simulink model "sf_demo"  (Simulink 6.4)
settings: Solver=FixedStepDiscrete  StartTime=0.0  StopTime=20  FixedStep=0.5  RelTol=1e-3
PreLoadFcn:
  | if exist('tl_preloadfcn','file'), tl_preloadfcn(gcs,95); end
PostLoadFcn:
  | if exist('tl_postloadfcn','file'), tl_postloadfcn(gcs,95); end
InitFcn:
  | if exist('tlds_start','file'), tlds_start(gcs); end
undefined symbols (not defined in the file or in its folder): built, Gain, in, Sum
libraries: tllib x18, simulink x1
PreSaveFcn:
  | if exist('tl_presavefcn','file'), tl_presavefcn(gcs); end
settings Model: LastModifiedBy=hilgers  ExtModeTrigMode=oneshot  ExtModeArmWhenConnect=off  BufferReuse=off  DS_PROJECTFILE=sf_demo.dd  TL_MAIN_DATA=struct('codeopt',struct('target',['Generic ANSI-C'],'optlevel',0,'sfbitfields',1,'limidentlength',1,'decimals',0,'assembler',1,'sections',1,'separatesearch',0,'cleancode',0,'optimizedbooltype',1,'inliningthreshold',5,'linebreaklimit',100,'stateactcodinglimit',5,'functionsfor64bitops',1,'globalbitfields',0,'sharefunctions',0,'noinitstozero',0,'keepsaturation',0,'extvarsharing',0,'outputstylefile','cconfig.xml','rootstylesheet','TL_CSourceCodeSS.xsl'),'frameopt',struct('exectime',1,'stacksize',1,'mexargs','','simconfig',['default EVM'],'targettimeout',1,'tcargs',''),'logopt',struct('plotinterval',0.1,'globalloggingmode',1),'date',732484.795619213,'asapscript','asap2_all_in_one','docscript','tldoc_default','maxnumsimulations',10,'export',struct('directory','.\export','sysfiles',1,'docfiles',0,'tools',0),'codecoveragelevel',0,'rtos',struct('enablemultirate',0,'currentrtos',['generic RTOS'],'autopriority',0,'autoinitalarm',1,'alarminitwithrestart',1,'alarmactivationkind',1,'alarmstartoffset',0))  TL_MODEL_COMMENT=This model implements a simple state machine.
settings DataIOCC: LimitDataPoints=off
settings OptimizationCC: BlockReduction=off  BooleanDataType=off  OptimizeBlockIOStorage=off  BufferReuse=off  ExpressionFolding=off  LocalBlockOutputs=off
settings DebuggingCC: SolverPrmCheckMsg=none  StrictBusMsg=None
settings HardwareCC: TargetEndianess=LittleEndian  TargetHWDeviceType=MATLAB Host  ProdEqTarget=off

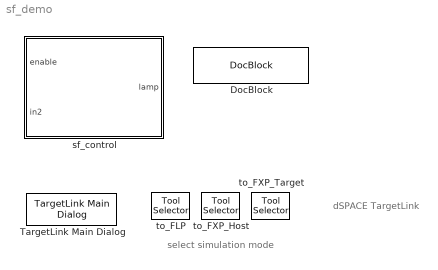
== system sf_demo ==
  note: select simulation mode
  note: dSPACE TargetLink
  DocBlock : simulink/Model-Wide Utilities/DocBlock  SystemSampleTime=-1  DocumentType=Text
  TargetLink Main Dialog : tllib/TargetLink Main Dialog  SystemSampleTime=-1  flp_block=none
  sf_control : Subsystem  Tag=TargetLink Simulation Frame
      settings: CopyFcn=if exist('tl_copyfcn','file'), tl_copyfcn(gcbh); end  NameChangeFcn=if exist('tl_framenamechangefcn','file'), tl_framenamechangefcn(gcbh); end  OpenFcn=if exist('open_tlsubsystem','file'), open_tlsubsystem(gcbh); end
      mask Type: TL_SimFrame
      mask Display: disp('TargetLink\nModel-\nin-the-loop\nmode')
  to_FLP : tllib/Tool Selector  Description=MIL\nmode  SystemSampleTime=-1  data=struct('date',732004.630535799)  flp_block=none
  to_FXP_Host : tllib/Tool Selector  Description=SIL\nmode  SystemSampleTime=-1  data=struct('date',732004.630535914)  flp_block=none
  to_FXP_Target : tllib/Tool Selector  Description=PIL\nmode  SystemSampleTime=-1  data=struct('date',732004.63053603)  flp_block=none

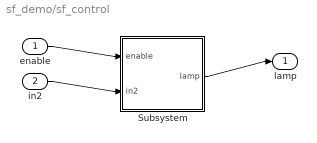
== system sf_demo/sf_control ==
  enable : Inport  PortDimensions=1  SampleTime=0.5  DataType=Specify via dialog  OutDataType=osc_int16
  in2 : Inport  Port=2  PortDimensions=1  SampleTime=0.5  DataType=Specify via dialog  OutDataType=osc_uint32
  Subsystem : Subsystem
      settings: OpenFcn=warndlg(get_param(gcb,'MaskHelp'),'Serious Warning');
      mask Type: TL_Enable
      mask Help: This subsystem keeps the TargetLink subsystem (subsystem with TargetLink blocks for production code generation), and is needed for the TargetLink simulation frame to work properly. DO NOT DELETE OR MODIFY IT!
  lamp : Outport
  wires:
  enable/1 -> Subsystem/1(enable)
  in2/1 -> Subsystem/2(in2)
  Subsystem/1(lamp) -> lamp/1

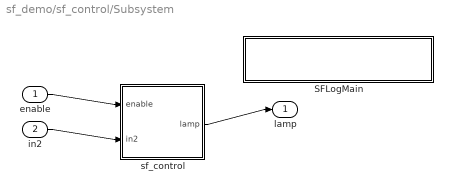
== system sf_demo/sf_control/Subsystem ==
  enable : Inport  PortDimensions=1  SampleTime=0.5  DataType=Specify via dialog  OutDataType=osc_int16
  in2 : Inport  Port=2  PortDimensions=1  SampleTime=0.5  DataType=Specify via dialog  OutDataType=osc_uint32
  SFLogMain : Subsystem
      mask Type: TL_StateflowLoggingMain
      mask Display:
      | plot([0 0 1 1 0 0 1 1 0],[0 1 1 0 0 0.05 0.05 0.95 0.95]);
      | disp('Stateflow Logging Main\nDO NOT DELETE')
  sf_control : Subsystem  Tag=MIL Subsystem  Description=a
      settings: CopyFcn=if exist('tl_copyfcn','file'), tl_copyfcn(gcbh); end  NameChangeFcn=if exist('tl_namechangefcn','file'), tl_namechangefcn(gcbh); end  DestroyFcn=if exist('update_tl_main_dlg','file'), update_tl_main_dlg('TL_subs_display'); end
  lamp : Outport
  wires:
  enable/1 -> sf_control/1(enable)
  in2/1 -> sf_control/2(in2)
  sf_control/1(lamp) -> lamp/1

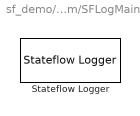
== system sf_demo/sf_control/Subsystem/SFLogMain ==
  Stateflow Logger : tllib/Extras/Stateflow Logger  data=struct('date',732004.630533947)  sflogparam=struct('charts',163,'sfblocks',{{'sf_demo/sf_control/Subsystem/sf_control/SF_TEST_B'}},'machines',162,'globallogopt',1,'modelname','sf_demo','debugmodeactive',1)  flp_block=tldummylib/Stateflow Logger

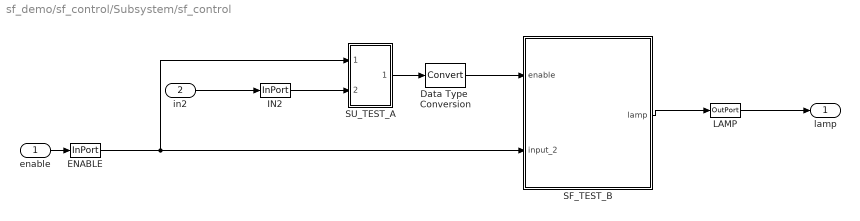
== system sf_demo/sf_control/Subsystem/sf_control ==
  enable : Inport  PortDimensions=1  SampleTime=0.5  DataType=Specify via dialog  OutDataType=osc_int16
      settings: CopyFcn=if exist('tl_check_ports','file'), tl_check_ports(gcbh); end  NameChangeFcn=if exist('tl_check_ports','file'), tl_check_ports(gcbh); end
  in2 : Inport  Port=2  PortDimensions=1  SampleTime=0.5  DataType=Specify via dialog  OutDataType=osc_uint32
      settings: CopyFcn=if exist('tl_check_ports','file'), tl_check_ports(gcbh); end  NameChangeFcn=if exist('tl_check_ports','file'), tl_check_ports(gcbh); end
  Data Type  Conversion : DataTypeConversion  OutDataTypeMode=Specify via dialog  OutDataType=osc_boolean  SaturateOnIntegerOverflow=on  RndMeth=Zero
  ENABLE : tllib/InPort  SystemSampleTime=-1  data=struct('logdata',struct('maxnumvals',4096,'plotchannels',1,'channels',1,'loggingmode',1),'output',struct('width',1,'name','$S_$B','unit','','type','Int8','offset',0,'max',1,'min',0,'freeze',1,'lsb',1,'arb',0,'class','FCN_ARG','address','','show',0,'description','','autoscalingmode',1,'lowerheadroom',1,'upperheadroom',1,'headroomunit','bit','variable','','scaling','','keepdatatype',1,'castoutput',0),'date',732458.608520498,'virtual',1,'message',struct('name','','component','','accessor',''),'scalingvalid',0)  flp_block=none
  IN2 : tllib/InPort  SystemSampleTime=-1  data=struct('logdata',struct('maxnumvals',4096,'plotchannels',1,'channels',1,'loggingmode',1),'output',struct('width',1,'name','$S_$B','unit','','type','Int8','offset',0,'max',1,'min',0,'freeze',1,'lsb',1,'arb',0,'class','FCN_ARG','address','','show',0,'description','','autoscalingmode',1,'lowerheadroom',1,'upperheadroom',1,'headroomunit','bit','variable','','scaling','','keepdatatype',1,'castoutput',0),'date',732463.617900926,'virtual',1,'message',struct('name','','component','','accessor',''),'scalingvalid',0)  flp_block=none
  LAMP : tllib/OutPort  SystemSampleTime=-1  data=struct('comment',struct('text','','placement',1),'logdata',struct('maxnumvals',inf,'plotchannels',1,'channels',1,'loggingmode',1),'output',struct('width',1,'name','$S_$B','unit','','type','Int8','offset',0,'max',1,'min',0,'freeze',1,'lsb',1,'arb',0,'class','FCN_RETURN','address','','checkmin',0,'checkmax',0,'show',0,'description','','autoscalingmode',1,'lowerheadroom',1,'upperheadroom',1,'headroomunit','bit','variable','','scaling','','keepdatatype',1,'castoutput',0),'date',732463.632425845,'virtual',1,'message',struct('name','','component',''),'scalingvalid',0)  flp_block=none
  SF_TEST_B : Stateflow chart
  SU_TEST_A : Subsystem  TreatAsAtomicUnit=on
  lamp : Outport
      settings: CopyFcn=if exist('tl_check_ports','file'), tl_check_ports(gcbh); end  NameChangeFcn=if exist('tl_check_ports','file'), tl_check_ports(gcbh); end
  wires:
  SF_TEST_B/1(lamp) -> LAMP/1
  LAMP/1 -> lamp/1
  enable/1 -> ENABLE/1
  in2/1 -> IN2/1
  ENABLE/1 -> SU_TEST_A/1(In1), SF_TEST_B/2(input_2)
  IN2/1 -> SU_TEST_A/2(In2)
  SU_TEST_A/1(Out1) -> Data Type  Conversion/1
  Data Type  Conversion/1 -> SF_TEST_B/1(enable)

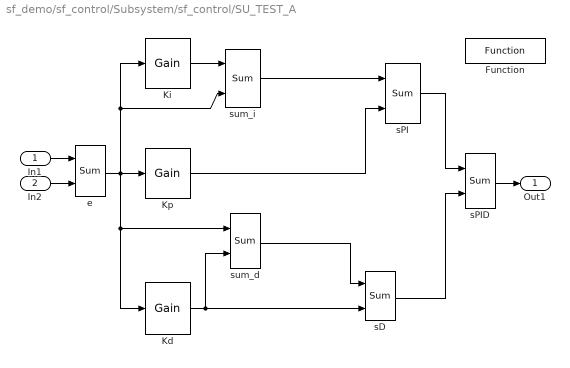
== system sf_demo/sf_control/Subsystem/sf_control/SU_TEST_A ==
  In1 : Inport  DataType=Specify via dialog  OutDataType=osc_int16
  In2 : Inport  Port=2  DataType=Specify via dialog  OutDataType=osc_uint32
  Function : tllib/Function  SystemSampleTime=-1  data=struct('revisionNumber',9,'description','','stepfunctionname','$S_$B','stepfunctionclass','default','forcerestartfunction',0,'restartfunctionname','RESTART_$S_$B','restartfunctionclass','default','forceinitfunction',0,'initfunctionname','INIT_$S_$B','initfunctionclass','default','forcetermfunction',0,'termfunctionname','TERM_$S_$B','termfunctionclass','default','subsystemid','default','forcereuse',0,'linkfile',0,'functionarglist',{{}},'unscaledarguments',0,'scalingpropagation',{{}},'incrcodegen',0,'ownedmodules',{{}},'destination','','addtestframe',0,'simmode',1,'codecomment','','codefile','','codecoveragelevel',0)  flp_block=tldummylib/Function
  Kd : tllib/Gain  Tag="Gain block of the dSPACE Fixed Point Code Generation Environment.      \\n                                                                       \\n signal is equal to the product of the input signal and the gain value:\\n\t\ty = G u"  SystemSampleTime=-1  data=struct('gain',struct('value','4','type','UInt8','lsb',2^-5,'offset',0,'min',NaN,'max',NaN,'arb',0,'freeze',1,'width',1,'scalar',0,'name','P_$D','class','CAL','address','','unit','','description','','tolerance',1,'variable','','scaling','','keepdatatype',1),'logdata',struct('maxnumvals',inf,'plotchannels',1,'channels',1,'loggingmode',3),'output',struct('type','Int16','lsb',2^-15,'offset',0,'max',NaN,'min',NaN,'checkmin',0,'checkmax',0,'arb',0,'freeze',1,'width',1,'name','$S_$B','show',0,'class','default','address','','unit','','description','','autoscalingmode',1,'lowerheadroom',1,'upperheadroom',1,'headroomunit','bit','variable','','scaling','','keepdatatype',1,'castoutput',0),'comment',struct('text','','placement',1),'date',732457.587188403,'scalingvalid',0)  gain=4  flp_block=built-in/Gain  help=Gain block of dSPACE TargetLink.\n\nOutput signal is equal to the product of the input signal and the gain value:\n\t\ty = G u
  Ki : tllib/Gain  SystemSampleTime=-1  data=struct('gain',struct('value','0.2','type','UInt8','lsb',2^-10,'offset',0,'min',NaN,'max',NaN,'arb',0,'freeze',1,'width',1,'scalar',0,'name','P_$D','class','CAL','address','','unit','','description','','tolerance',1,'variable','','scaling','','keepdatatype',1),'logdata',struct('maxnumvals',inf,'plotchannels',[],'channels',1,'loggingmode',3),'output',struct('type','Int16','lsb',2^-20,'offset',0,'max',NaN,'min',NaN,'checkmin',0,'checkmax',0,'arb',0,'freeze',1,'width',1,'name','$S_$B','show',0,'class','default','address','','unit','','description','','autoscalingmode',1,'lowerheadroom',1,'upperheadroom',1,'headroomunit','bit','variable','','scaling','','keepdatatype',1,'castoutput',0),'comment',struct('text','','placement',1),'date',732457.586778785,'scalingvalid',0)  gain=0.2  flp_block=built-in/Gain  help=Gain block of dSPACE TargetLink.\n\nOutput signal is equal to the product of the input signal and the gain value:\n\t\ty = G u
  Kp : tllib/Gain  Tag="Gain block of the dSPACE Fixed Point Code Generation Environment.      \\n                                                                       \\n signal is equal to the product of the input signal and the gain value:\\n\t\ty = G u"  SystemSampleTime=-1  data=struct('gain',struct('value','1.2','type','UInt8','lsb',2^-7,'offset',0,'min',NaN,'max',NaN,'arb',0,'freeze',1,'width',1,'scalar',0,'name','P_$D','class','CAL','address','','unit','','description','','tolerance',1,'variable','','scaling','','keepdatatype',1),'logdata',struct('maxnumvals',inf,'plotchannels',[],'channels',1,'loggingmode',3),'output',struct('type','Int16','lsb',2^-17,'offset',0,'max',NaN,'min',NaN,'checkmin',0,'checkmax',0,'arb',0,'freeze',1,'width',1,'name','$S_$B','show',0,'class','default','address','','unit','','description','','autoscalingmode',1,'lowerheadroom',1,'upperheadroom',1,'headroomunit','bit','variable','','scaling','','keepdatatype',1,'castoutput',0),'comment',struct('text','','placement',1),'date',732457.587011169,'scalingvalid',0)  gain=1.2  flp_block=built-in/Gain  help=Gain block of dSPACE TargetLink.\n\nOutput signal is equal to the product of the input signal and the gain value:\n\t\ty = G u
  e : tllib/Sum  data=struct('logdata',struct('maxnumvals',inf,'plotchannels',1,'channels',1,'loggingmode',1),'output',struct('type','Int16','lsb',2^-18,'offset',0,'max',NaN,'min',NaN,'checkmin',1,'checkmax',1,'arb',0,'freeze',1,'width',1,'name','$S_$B','show',0,'class','default','address','','unit','','description','','autoscalingmode',1,'lowerheadroom',1,'upperheadroom',1,'headroomunit','bit','variable','','scaling','','keepdatatype',1,'castoutput',0),'inputs','+-','comment',struct('text','','placement',1),'date',732457.596463576,'scalingvalid',0)  flp_block=built-in/Sum  help=Sum block of dSPACE TargetLink.\n\nOutput signal is equal to the sum of the input signals.\nThe list of signs is specified according to conventions for Simulink Sum blocks.
  sD : tllib/Sum  Tag="Sum block of the dSPACE Fixed Point Code Generation Environment.\\n                                                                \\nOutput signal is equal to the sum of the two input signals:     \\n                                                                \\n\t\ty = u1 - u2"  data=struct('logdata',struct('maxnumvals',inf,'plotchannels',1,'channels',1,'loggingmode',3),'output',struct('type','Int16','lsb',2^-15,'offset',0,'max',NaN,'min',NaN,'checkmin',0,'checkmax',0,'arb',0,'freeze',1,'width',1,'name','$S_$B','show',0,'class','default','address','','unit','','description','','autoscalingmode',1,'lowerheadroom',1,'upperheadroom',1,'headroomunit','bit','variable','','scaling','','keepdatatype',1,'castoutput',0),'inputs','++','comment',struct('text','','placement',1),'date',732004.633502326,'scalingvalid',0)  flp_block=built-in/Sum  help=Sum block of dSPACE TargetLink.\n\nOutput signal is equal to the sum of the input signals.\nThe list of signs is specified according to conventions for Simulink Sum blocks.
  sPI : tllib/Sum  Tag="Sum block of the dSPACE Fixed Point Code Generation Environment.\\n                                                                \\nOutput signal is equal to the sum of the two input signals:     \\n                                                                \\n\t\ty = u1 - u2"  data=struct('logdata',struct('maxnumvals',inf,'plotchannels',[],'channels',1,'loggingmode',3),'output',struct('type','Int16','lsb',2^-17,'offset',0,'max',NaN,'min',NaN,'checkmin',0,'checkmax',0,'arb',0,'freeze',1,'width',1,'name','$S_$B','show',0,'class','default','address','','unit','','description','','autoscalingmode',1,'lowerheadroom',1,'upperheadroom',1,'headroomunit','bit','variable','','scaling','','keepdatatype',1,'castoutput',0),'inputs','++','comment',struct('text','','placement',1),'date',732004.633503032,'scalingvalid',0)  flp_block=built-in/Sum  help=Sum block of dSPACE TargetLink.\n\nOutput signal is equal to the sum of the input signals.\nThe list of signs is specified according to conventions for Simulink Sum blocks.
  sPID : tllib/Sum  data=struct('logdata',struct('maxnumvals',inf,'plotchannels',1,'channels',1,'loggingmode',3),'output',struct('type','Int16','lsb',2^-15,'offset',0,'max',NaN,'min',NaN,'checkmin',0,'checkmax',0,'arb',0,'freeze',1,'width',1,'name','$S_$B','show',0,'class','default','address','','unit','','description','','autoscalingmode',1,'lowerheadroom',1,'upperheadroom',1,'headroomunit','bit','variable','','scaling','','keepdatatype',1,'castoutput',0),'inputs','++','comment',struct('text','','placement',1),'date',732458.608752708,'scalingvalid',0)  flp_block=built-in/Sum  help=Sum block of dSPACE TargetLink.\n\nOutput signal is equal to the sum of the input signals.\nThe list of signs is specified according to conventions for Simulink Sum blocks.
  sum_d : tllib/Sum  data=struct('logdata',struct('maxnumvals',inf,'plotchannels',[],'channels',1,'loggingmode',3),'output',struct('type','Int16','lsb',2^-15,'offset',0,'max',NaN,'min',NaN,'checkmin',0,'checkmax',0,'arb',0,'freeze',1,'width',1,'name','$S_$B','show',0,'class','default','address','','unit','','description','','autoscalingmode',1,'lowerheadroom',1,'upperheadroom',1,'headroomunit','bit','variable','','scaling','','keepdatatype',1,'castoutput',0),'inputs','+-','comment',struct('text','','placement',1),'date',732004.633504421,'scalingvalid',0)  flp_block=built-in/Sum  help=Sum block of dSPACE TargetLink.\n\nOutput signal is equal to the sum of the input signals.\nThe list of signs is specified according to conventions for Simulink Sum blocks.
  sum_i : tllib/Sum  Tag="Sum block of the dSPACE Fixed Point Code Generation Environment.\\n                                                                \\nOutput signal is equal to the sum of the two input signals:     \\n                                                                \\n\t\ty = u1 - u2"  data=struct('logdata',struct('maxnumvals',inf,'plotchannels',[],'channels',1,'loggingmode',3),'output',struct('type','Int16','lsb',2^-19,'offset',0,'max',NaN,'min',NaN,'checkmin',0,'checkmax',0,'arb',0,'freeze',1,'width',1,'name','$S_$B','show',0,'class','default','address','','unit','','description','','autoscalingmode',1,'lowerheadroom',1,'upperheadroom',1,'headroomunit','bit','variable','','scaling','','keepdatatype',1,'castoutput',0),'inputs','+-','comment',struct('text','','placement',1),'date',732464.693850544,'scalingvalid',0)  flp_block=built-in/Sum  help=Sum block of dSPACE TargetLink.\n\nOutput signal is equal to the sum of the input signals.\nThe list of signs is specified according to conventions for Simulink Sum blocks.
  Out1 : Outport
  wires:
  Kd/1 -> sum_d/2, sD/2
  sD/1 -> sPID/2
  sum_d/1 -> sD/1
  sPI/1 -> sPID/1
  sum_i/1 -> sPI/1
  Ki/1 -> sum_i/1
  Kp/1 -> sPI/2
  e/1 -> Kp/1, Ki/1, sum_i/2, Kd/1, sum_d/1
  In1/1 -> e/1
  In2/1 -> e/2
  sPID/1 -> Out1/1

== stateflow chart sf_control/Subsystem/sf_control/SF_TEST_B ==
  settings: sampleTime=1
  state do_blink
    state BLINKER_ON/
      entry:lamp=1;
    state BLINKER_OFF
      entry: lamp = 0;
    BLINKER_ON -> BLINKER_OFF
    BLINKER_OFF -> BLINKER_ON
  state OFF
    entry: lamp = 0;
  (default) -> OFF
  OFF -> BLINKER_ON : [enable == 1]
  do_blink -> OFF : [enable==0]
  data: enable input osc_boolean; lamp output osc_int32; input_2 input osc_int16
